simulink model "new_anf"  (R2017b)
settings: Solver=ode23t  StartTime=0.0  StopTime=0.5  MaxStep=1e-4  RelTol=1e-3
libraries: powerlib x22
settings Model: Creator=Abhishek  LastModifiedBy=Kalpit

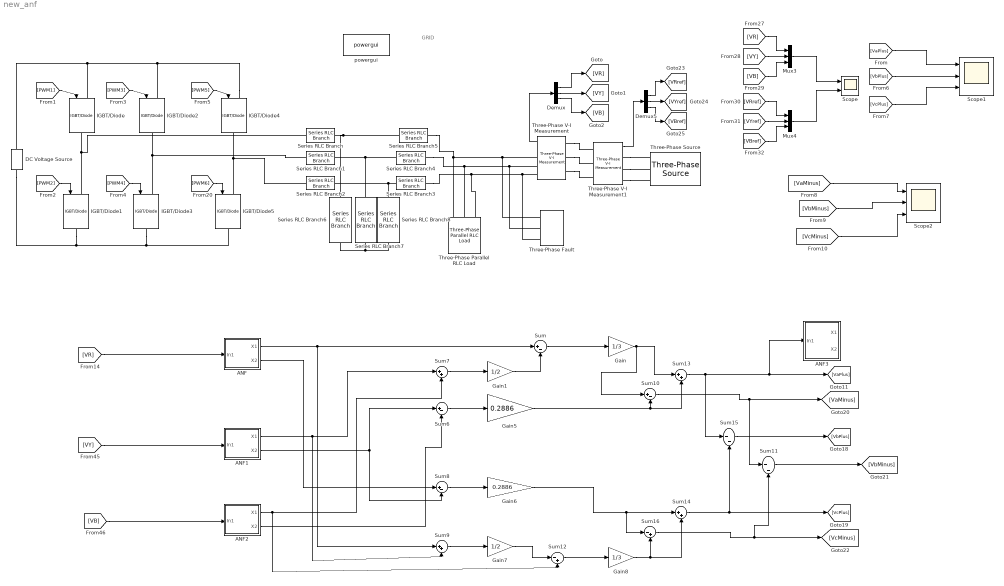
== system new_anf ==
  note: GRID
  ANF : Subsystem
  ANF1 : Subsystem
  ANF2 : Subsystem
  ANF3 : Subsystem
  DC Voltage Source : powerlib/Electrical Sources/DC Voltage Source  Amplitude=600  Measurements=None
  Demux : Demux  Outputs=3
  Demux5 : Demux  Outputs=3
  Gain : Gain  Gain=1/3
  Gain1 : Gain  Gain=1/2
  Gain5 : Gain  Gain=0.2886
  Gain6 : Gain  Gain=0.2886
  Gain7 : Gain  Gain=1/2
  Gain8 : Gain  Gain=1/3
  IGBT/Diode{,1..5} (6 alike) : powerlib/Power Electronics/IGBT//Diode  Ron=1e-3  Rs=1e5  Cs=inf  Measurements=off
  Mux3 : Mux  Inputs=3
  Mux4 : Mux  Inputs=3
  Scope : Scope  NumInputPorts=2
  Scope1 : Scope  NumInputPorts=3
  Scope2 : Scope  NumInputPorts=3
  Series RLC Branch{,1..5} (6 alike) : powerlib/Elements/Series RLC Branch  LConnTagsString=__new0  RConnTagsString=__new0  BranchType=L  Resistance=1  Inductance=800e-3  SetiL0=off  InitialCurrent=0  Capacitance=1e-6  Setx0=off  InitialVoltage=0  Measurements=None
  Series RLC Branch6 : powerlib/Elements/Series RLC Branch  LConnTagsString=__new0  RConnTagsString=__new0  BranchType=C  Resistance=1  Inductance=500e-6  SetiL0=off  InitialCurrent=0  Capacitance=30e-6  Setx0=off  InitialVoltage=0  Measurements=None
  Series RLC Branch7 : powerlib/Elements/Series RLC Branch  LConnTagsString=__new0  RConnTagsString=__new0  BranchType=C  Resistance=1  Inductance=500e-6  SetiL0=off  InitialCurrent=0  Capacitance=30e-6  Setx0=off  InitialVoltage=0  Measurements=None
  Series RLC Branch8 : powerlib/Elements/Series RLC Branch  LConnTagsString=__new0  RConnTagsString=__new0  BranchType=C  Resistance=1  Inductance=500e-6  SetiL0=off  InitialCurrent=0  Capacitance=30e-6  Setx0=off  InitialVoltage=0  Measurements=None
  Sum{,6,8,10} (4 alike) : Sum  Inputs=|+-
  Sum11 : Sum  Inputs=|--
  Sum12 : Sum  Inputs=|-+
  Sum{7,9,13..14} (4 alike) : Sum  Inputs=|++
  Sum15 : Sum  Inputs=|--
  Sum16 : Sum  Inputs=|-+
  Three-Phase Parallel RLC Load : powerlib/Elements/Three-Phase Parallel RLC Load  LConnTagsString=A|B|C  Configuration=Delta  NominalVoltage=230  Vabc=[1e3 1e3 1e3]  Vabcp=[1e3 1e3 1e3]  NominalFrequency=50  UnbalancedPower=off  ActivePower=60e6  InductivePower=40e6  CapacitivePower=0  Pabc=[10e3 9e3 11e3]  QLabc=[100 90 110]  QCabc=[100 90 110]  Pabcp=[10e3 9e3 11e3]  QLabcp=[100 90 110]  QCabcp=[100 90 110]  Measurements=None  LoadType=constant PQ
  Three-Phase V-I Measurement : powerlib/Measurements/Three-Phase V-I Measurement  VoltageMeasurement=phase-to-phase  SetLabelV=off  LabelV=Vabc  Vpu=off  VpuLL=off  CurrentMeasurement=yes  SetLabelI=off  LabelI=Iabc  Ipu=off  Pbase=100e3  Vbase=230  OutputType=Complex  PhasorSimulation=off  PSBequivalent=0
  Three-Phase V-I Measurement1 : powerlib/Measurements/Three-Phase V-I Measurement  VoltageMeasurement=phase-to-phase  SetLabelV=off  LabelV=Vabc  Vpu=off  VpuLL=off  CurrentMeasurement=no  SetLabelI=off  LabelI=Iabc  Ipu=off  Pbase=100e6  Vbase=500e3  OutputType=Complex  PhasorSimulation=off  PSBequivalent=0
  Three-Phase Fault : powerlib/Elements/Three-Phase Fault  InitialStates=1  FaultA=on  FaultB=on  FaultC=off  GroundFault=on  SwitchTimes=0.25  External=off  SwitchStatus=NaN  FaultResistance=1e-6  GroundResistance=1e-6  SnubberResistance=1e6  SnubberCapacitance=inf  Measurements=None
  Three-Phase Source : powerlib/Electrical Sources/Three-Phase Source  InternalConnection=Yg  VoltagePhases=off  Voltage=415  PhaseAngle=0  Voltage_phases=[25e3 25e3 25e3]/sqrt(3)  PhaseAngles_phases=[0 -120 +120]  Frequency=50  NonIdealSource=on  SpecifyImpedance=off  Resistance=.001e-3  Inductance=.001e-9  ShortCircuitLevel=100e6  BaseVoltage=415  XRratio=7  BusType=swing  Pref=10e3  Qref=0  Prefabc=[10e3, 10e3, 10e3]  Qrefabc=[0, 0, 0]  Qmin=-inf  Qmax=inf
  powergui : powerlib/powergui  Priority=1  SimulationMode=Discrete  SampleTime=1e-6  frequency=60  Iterations=50  frequencyindice=0  Pbase=100e6  ErrMax=1e-4  UnitsV=kV  UnitsW=MW  buscounter=0  FunctionMessages=off  echomessages=off  EnableUseOfTLC=off  CurrentSourceSwitches=off  DisableSnubberDevices=off  DisableRonSwitches=off  DisableVfSwitches=off  DisplayEquations=off  SolverType=Tustin/Backward Euler (TBE)  Interpol=off  ExternalGateDelay=off  methode=off  Ts=100  x0status=blocks  SPID=on  SwTol=0  HookPort=off  RestoreLinks=warning  ResistiveCurrentMeasurement=off  Frange=[0:2:500]  Ylog=off  Xlog=on  ShowGrid=off  save=off  variable=ZData  structure=0  ZoomFFT=off  StartTime=0.0  cycles=1  DisplayStyle=1  fundamental=60  FreqAxis=off  MaxFrequency=1000  frequencyindicesteady=1  RmsSteady=1  display=off
  wires:
  [VB] -> Mux3/3
  [VY] -> Mux3/2
  [VR] -> Mux3/1
  Mux3/1 -> Scope/1
  [VYref] -> Mux4/2
  Mux4/1 -> Scope/2
  [VRref] -> Mux4/1
  [VBref] -> Mux4/3
  Demux5/2 -> [VYref]
  Demux5/3 -> [VBref]
  Demux5/1 -> [VRref]
  Three-Phase V-I Measurement1/1 -> Demux5/1
  [PWM5] -> IGBT/Diode4/1
  [PWM3] -> IGBT/Diode2/1
  [PWM1] -> IGBT/Diode/1
  [PWM4] -> IGBT/Diode3/1
  [PWM2] -> IGBT/Diode1/1
  [PWM6] -> IGBT/Diode5/1
  Three-Phase V-I Measurement/1 -> Demux/1
  Demux/2 -> [VY]
  Demux/3 -> [VB]
  Sum12/1 -> Gain8/1
  Gain/1 -> Sum10/1, Sum13/1
  Sum7/1 -> Gain1/1
  Sum6/1 -> Gain5/1
  Gain7/1 -> Sum12/1
  Sum14/1 -> [VcPlus], Sum15/2
  ANF1/1(X1) -> Sum9/2, Sum7/1
  Sum/1 -> Gain/1
  Gain8/1 -> Sum16/2, Sum14/2
  Sum11/1 -> [VbMinus]
  Gain5/1 -> Sum10/2, Sum13/2
  Sum10/1 -> Sum11/1, [VaMinus]
  Sum13/1 -> Sum15/1, ANF3/1(In1), [VaPlus]
  ANF/1(X1) -> Sum9/1, Sum/1
  ANF2/1(X1) -> Sum12/2, Sum7/2
  ANF1/2(X2) -> Sum6/1, Sum8/2
  Sum9/1 -> Gain7/1
  Sum15/1 -> [VbPlus]
  Sum8/1 -> Gain6/1
  Gain1/1 -> Sum/2
  Gain6/1 -> Sum16/1, Sum14/1
  ANF2/2(X2) -> Sum6/2
  ANF/2(X2) -> Sum8/1
  Sum16/1 -> Sum11/2, [VcMinus]
  [VB] -> ANF2/1(In1)
  [VR] -> ANF/1(In1)
  [VY] -> ANF1/1(In1)
  [VcPlus] -> Scope1/3
  [VbPlus] -> Scope1/2
  [VaPlus] -> Scope1/1
  [VcMinus] -> Scope2/3
  [VaMinus] -> Scope2/1
  [VbMinus] -> Scope2/2
  Demux/1 -> [VR]
  connections:
  IGBT/Diode/RConn1 -- Series RLC Branch/LConn1 -- IGBT/Diode1/LConn1
  Series RLC Branch6/RConn1 -- Series RLC Branch7/RConn1 -- Series RLC Branch8/RConn1
  Three-Phase V-I Measurement1/RConn1 -- Three-Phase Source/RConn1
  Three-Phase V-I Measurement1/RConn2 -- Three-Phase Source/RConn2
  Three-Phase V-I Measurement1/RConn3 -- Three-Phase Source/RConn3
  IGBT/Diode4/LConn1 -- IGBT/Diode/LConn1 -- DC Voltage Source/RConn1 -- IGBT/Diode2/LConn1
  IGBT/Diode5/RConn1 -- DC Voltage Source/LConn1 -- IGBT/Diode1/RConn1 -- IGBT/Diode3/RConn1
  Three-Phase V-I Measurement/LConn2 -- Three-Phase V-I Measurement1/LConn2
  Three-Phase V-I Measurement/LConn1 -- Three-Phase V-I Measurement1/LConn1
  Three-Phase V-I Measurement/LConn3 -- Three-Phase V-I Measurement1/LConn3
  Series RLC Branch5/RConn1 -- Three-Phase Parallel RLC Load/LConn1 -- Three-Phase Fault/LConn1 -- Three-Phase V-I Measurement/RConn1
  Series RLC Branch4/RConn1 -- Three-Phase Parallel RLC Load/LConn2 -- Three-Phase Fault/LConn2 -- Three-Phase V-I Measurement/RConn2
  Series RLC Branch3/RConn1 -- Three-Phase Parallel RLC Load/LConn3 -- Three-Phase Fault/LConn3 -- Three-Phase V-I Measurement/RConn3
  Series RLC Branch3/LConn1 -- Series RLC Branch8/LConn1 -- Series RLC Branch2/RConn1
  Series RLC Branch4/LConn1 -- Series RLC Branch7/LConn1 -- Series RLC Branch1/RConn1
  Series RLC Branch5/LConn1 -- Series RLC Branch6/LConn1 -- Series RLC Branch/RConn1
  IGBT/Diode3/LConn1 -- Series RLC Branch1/LConn1 -- IGBT/Diode2/RConn1
  IGBT/Diode5/LConn1 -- Series RLC Branch2/LConn1 -- IGBT/Diode4/RConn1

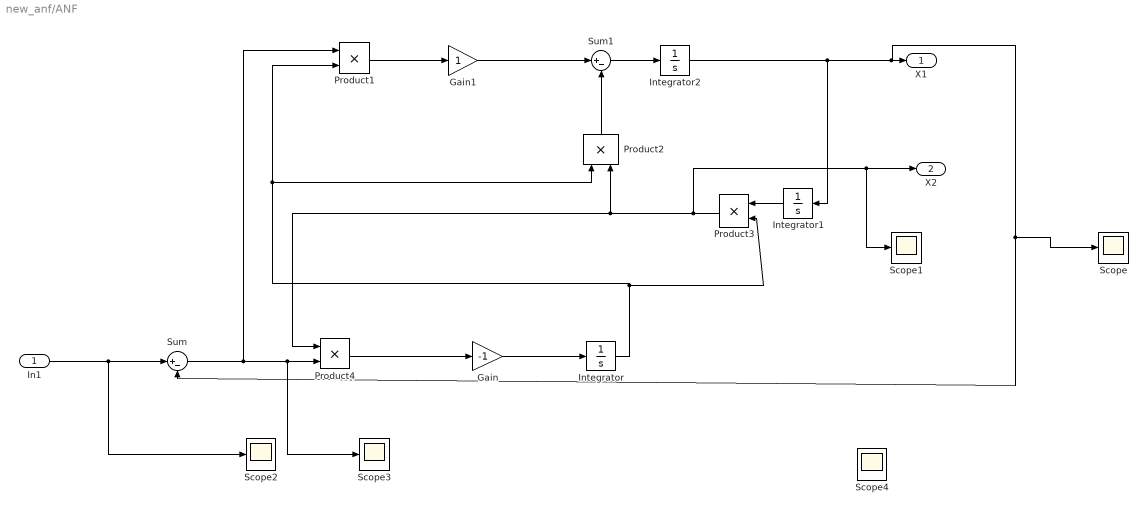
== system new_anf/ANF ==
  In1 : Inport
  Gain : Gain  Gain=-1
  Gain1 : Gain
  Integrator : Integrator  InitialCondition=100*pi
  Integrator1 : Integrator
  Integrator2 : Integrator
  Product{1..4} (4 alike) : Product
  Scope{,1..4} (5 alike) : Scope
  Sum : Sum  Inputs=|+-
  Sum1 : Sum  Inputs=|+-
  X1 : Outport
  X2 : Outport  Port=2
  wires:
  Sum1/1 -> Integrator2/1
  Sum/1 -> Product1/1, Scope3/1, Product4/2
  Product4/1 -> Gain/1
  In1/1 -> Scope2/1, Sum/1
  Integrator1/1 -> Product3/1
  Integrator2/1 -> Scope/1, Sum/2, X1/1, Integrator1/1
  Integrator/1 -> Product3/2, Product2/1, Product1/2
  Product3/1 -> Scope1/1, X2/1, Product4/1, Product2/2
  Product1/1 -> Gain1/1
  Product2/1 -> Sum1/2
  Gain/1 -> Integrator/1
  Gain1/1 -> Sum1/1

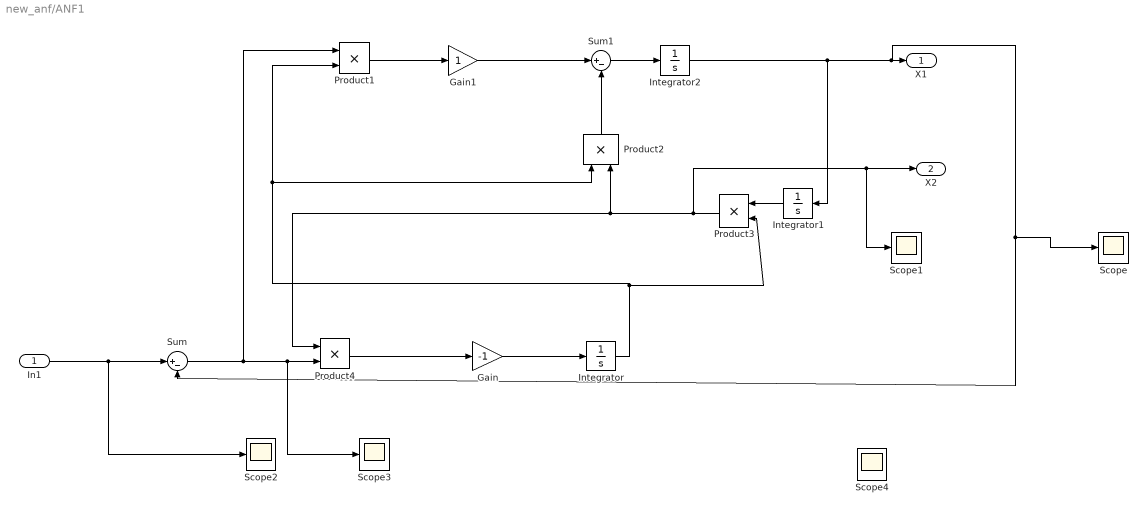
== system new_anf/ANF1 ==
  In1 : Inport
  Gain : Gain  Gain=-1
  Gain1 : Gain
  Integrator : Integrator  InitialCondition=100*pi
  Integrator1 : Integrator
  Integrator2 : Integrator
  Product{1..4} (4 alike) : Product
  Scope{,1..4} (5 alike) : Scope
  Sum : Sum  Inputs=|+-
  Sum1 : Sum  Inputs=|+-
  X1 : Outport
  X2 : Outport  Port=2
  wires:
  Gain1/1 -> Sum1/1
  Gain/1 -> Integrator/1
  Product2/1 -> Sum1/2
  Product1/1 -> Gain1/1
  Product3/1 -> Product2/2, Product4/1, X2/1, Scope1/1
  Integrator/1 -> Product1/2, Product2/1, Product3/2
  Integrator2/1 -> Integrator1/1, X1/1, Sum/2, Scope/1
  Integrator1/1 -> Product3/1
  In1/1 -> Sum/1, Scope2/1
  Product4/1 -> Gain/1
  Sum/1 -> Product4/2, Scope3/1, Product1/1
  Sum1/1 -> Integrator2/1

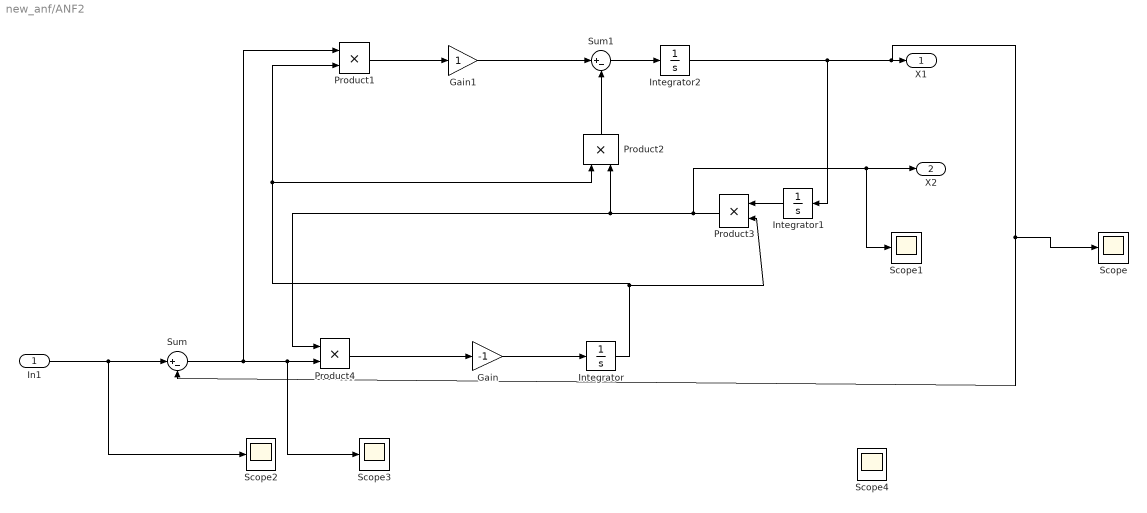
== system new_anf/ANF2 ==
  In1 : Inport
  Gain : Gain  Gain=-1
  Gain1 : Gain
  Integrator : Integrator  InitialCondition=100*pi
  Integrator1 : Integrator
  Integrator2 : Integrator
  Product{1..4} (4 alike) : Product
  Scope{,1..4} (5 alike) : Scope
  Sum : Sum  Inputs=|+-
  Sum1 : Sum  Inputs=|+-
  X1 : Outport
  X2 : Outport  Port=2
  wires:
  Sum1/1 -> Integrator2/1
  Sum/1 -> Product1/1, Scope3/1, Product4/2
  Product4/1 -> Gain/1
  In1/1 -> Scope2/1, Sum/1
  Integrator1/1 -> Product3/1
  Integrator2/1 -> Scope/1, Sum/2, X1/1, Integrator1/1
  Integrator/1 -> Product3/2, Product2/1, Product1/2
  Product3/1 -> Scope1/1, X2/1, Product4/1, Product2/2
  Product1/1 -> Gain1/1
  Product2/1 -> Sum1/2
  Gain/1 -> Integrator/1
  Gain1/1 -> Sum1/1

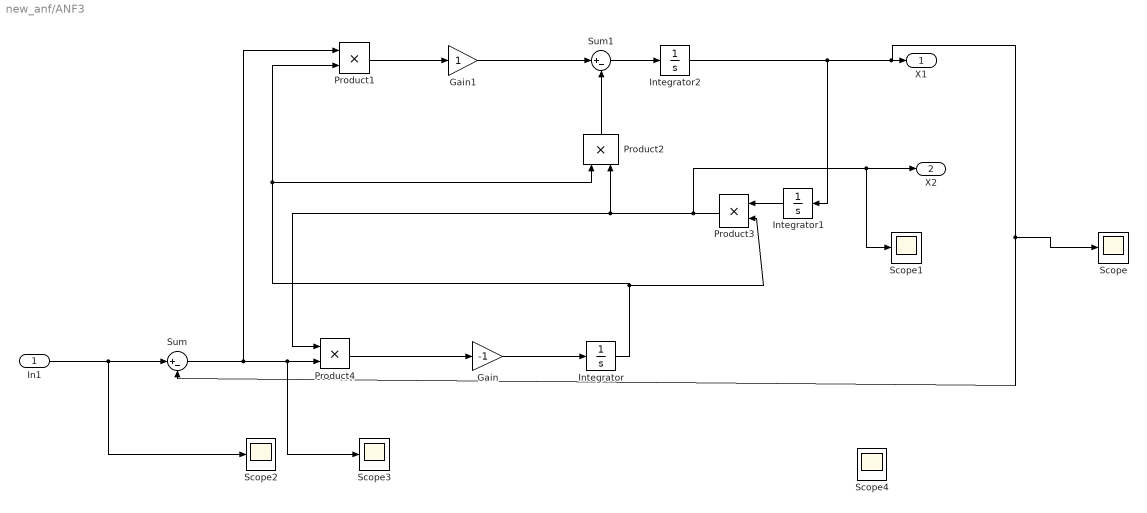
== system new_anf/ANF3 ==
  In1 : Inport
  Gain : Gain  Gain=-1
  Gain1 : Gain
  Integrator : Integrator  InitialCondition=100*pi
  Integrator1 : Integrator
  Integrator2 : Integrator
  Product{1..4} (4 alike) : Product
  Scope{,1..4} (5 alike) : Scope
  Sum : Sum  Inputs=|+-
  Sum1 : Sum  Inputs=|+-
  X1 : Outport
  X2 : Outport  Port=2
  wires:
  Sum1/1 -> Integrator2/1
  Sum/1 -> Product1/1, Scope3/1, Product4/2
  Product4/1 -> Gain/1
  In1/1 -> Scope2/1, Sum/1
  Integrator1/1 -> Product3/1
  Integrator2/1 -> Scope/1, Sum/2, X1/1, Integrator1/1
  Integrator/1 -> Product3/2, Product2/1, Product1/2
  Product3/1 -> Scope1/1, X2/1, Product4/1, Product2/2
  Product1/1 -> Gain1/1
  Product2/1 -> Sum1/2
  Gain/1 -> Integrator/1
  Gain1/1 -> Sum1/1
